simulink model "DA40_Flight_Model"  (R2023a)
settings: Solver=FixedStepAuto  StartTime=Start_Time  StopTime=End_Time  FixedStep=Time_Step  RelTol=1e-3
undefined symbols (not defined in the file or in its folder): BSFC_LUT, dayofyear, Earth, Initial_X, lookaheadDist, PowerFactor_LUT, STGeometry, Vehicle, waypoints, WGS84
libraries: slpidlib x8, simulink_extras x3, aerolibatmos2 x2, mspsensorlib x2, aerolibtransform2 x2, simulink x1, aerolibwind2 x1, uavalgslib x1
(part 1 of 3)
settings Model: Creator=izc0018  LastModifiedBy=noahm
settings DebuggingCC: AlgebraicLoopMsg=none  UnconnectedInputMsg=warning  UnconnectedOutputMsg=warning  UnconnectedLineMsg=warning
settings HardwareCC: ProdBitPerLong=64  ProdLargestAtomicFloat=None  ProdHWDeviceType=AMD->Athlon 64
settings ModelReferenceCC: EnableRefExpFcnMdlSchedulingChecks=on  ModelReferenceMinAlgLoopOccurrences=on
settings RTWCC: DLArmComputeVersion=19.05

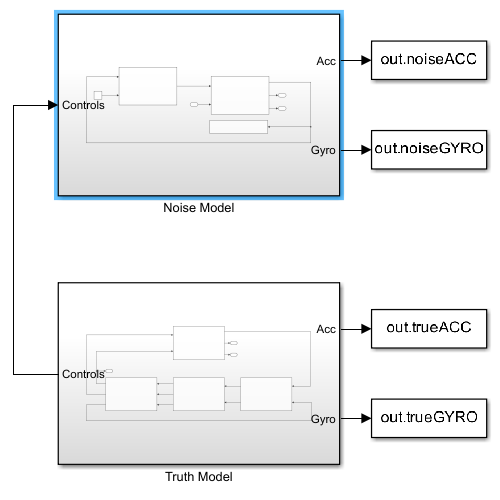
[thumbnail: Simulink's stored preview of the top-level diagram]
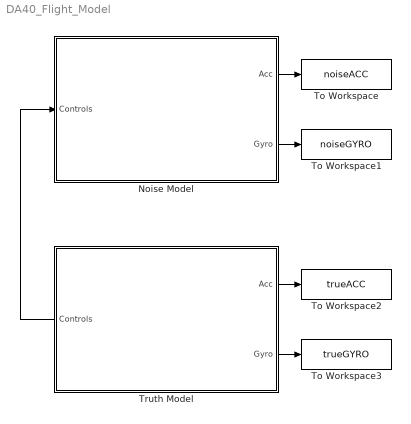
== system DA40_Flight_Model ==
  Noise Model : Subsystem
  To Workspace : ToWorkspace  VariableName=noiseACC  SaveFormat=Timeseries  SampleTime=-1
  To Workspace1 : ToWorkspace  VariableName=noiseGYRO  SaveFormat=Timeseries  SampleTime=-1
  To Workspace2 : ToWorkspace  VariableName=trueACC  SaveFormat=Timeseries  SampleTime=-1
  To Workspace3 : ToWorkspace  VariableName=trueGYRO  SaveFormat=Timeseries  SampleTime=-1
  Truth Model : Subsystem
      settings: PortSchema="{\"entries\":[{\"content\":{\"sides\":[{\"content\":{\"connectorIds\":[\"Out3\"]},\"type\":\"ConnectorPlacement.EquallySpacedRectSide\",\"uuid\":\"8eb98788-9771-4626-a3f5-af2a13caf3fb\"},{\"content\":{\"connectorIds\":[\"Out1\",\"Out2\"],\"side\":\"RIGHT\"},\"type\":\"ConnectorPlacement.EquallySpacedRectSide\",\"uuid\":\"345bd972-994d-44f9-8c5e-03b63b24e0ec\"},{\"content\":{\"side\":\"TOP\"},\"type\":\"ConnectorPlacement.EquallySpacedRectSide\",\"uuid\":\"1da6d2e0-f9fd-4d97-b889-7f9e1c209230\"}]},\"type\":\"ConnectorPlacement.EquallySpacedConnector\",\"uuid\":\"7d2beb0e-411b-47ae-aba6-e2acf08d65c2\"}],\"packageUris\":[\"http://schema.mathworks.com/mf0/Connector/R2020b\"],\"version\":\"1.0\"}"
  wires:
  Truth Model/3(Controls) -> Noise Model/1(Controls)
  Noise Model/1(Acc) -> To Workspace/1
  Noise Model/2(Gyro) -> To Workspace1/1
  Truth Model/1(Acc) -> To Workspace2/1
  Truth Model/2(Gyro) -> To Workspace3/1

== system DA40_Flight_Model/Noise Model ==
  Controls : Inport
  Band-Limited White Noise3 : simulink/Sources/Band-Limited White Noise  Cov=500  Ts=30  seed=1
  Environment : Subsystem
  Navigation : Subsystem
  Send To Workspace : Subsystem
  Acc : Outport
  Gyro : Outport  Port=2
  wires:
  Environment/1(Atmos) -> Navigation/1(Atmosphere)
  Navigation/1(States) -> Environment/1(States), Send To Workspace/1(States)
  Band-Limited White Noise3/1 -> Environment/2(Wind Model)
  Controls/1 -> Navigation/2(Controls)
  Navigation/2(Acc) -> Acc/1
  Navigation/3(Gyro) -> Gyro/1

== system DA40_Flight_Model/Truth Model ==
  Control : Subsystem
  Environment : Subsystem
  Guidance : Subsystem
  Navigation1 : Subsystem
  Acc : Outport
  Gyro : Outport  Port=2
  Controls : Outport  Port=3
  wires:
  Control/1(Controls) -> Navigation1/2(Controls), Controls/1
  Guidance/1(Commands) -> Control/1(Commands)
  Guidance/2(States Out) -> Control/2(States)
  Guidance/3(Atmos) -> Control/3(Atmos)
  Environment/1(States Out) -> Guidance/1(States)
  Environment/2(Atmos) -> Guidance/2(Atmosphere)
  Control/3(LLA) -> Environment/2(LLA)
  Control/2(Atmosphere) -> Navigation1/1(Atmosphere)
  Navigation1/1(States) -> Environment/1(States)
  Navigation1/2(Acc) -> Acc/1
  Navigation1/3(Gyro) -> Gyro/1

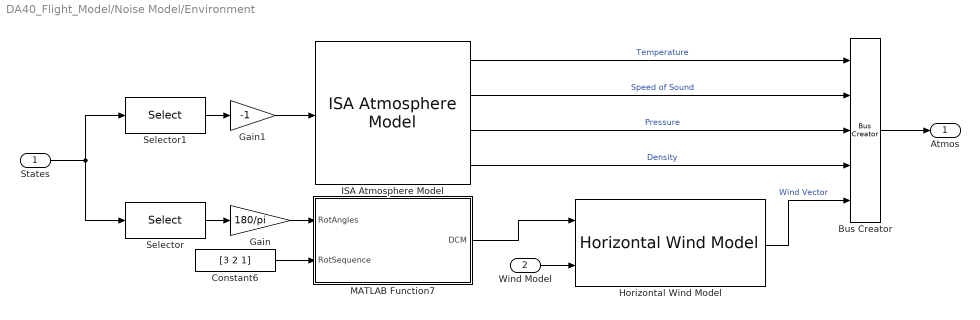
== system DA40_Flight_Model/Noise Model/Environment ==
  States : Inport
  Wind Model : Inport  Port=2
  Bus Creator : BusCreator  Inputs=5
  Constant6 : Constant  Value=[3 2 1]
  Gain : Gain  Gain=180/pi
  Gain1 : Gain  Gain=-1
  Horizontal Wind Model : aerolibwind2/Horizontal Wind Model  units=Metric (MKS)  Vw_source=External  Vwind=0  W_source=Internal  Wdeg=0
  ISA Atmosphere Model : aerolibatmos2/ISA Atmosphere Model  custom=off  g=9.80665  gamma=1.4  R=287.0531  L=0.0065  h_trop=11000  h_strat=20000  rho0=1.225  P0=101325  T0=288.15  h0=0
  MATLAB Function7 : MATLAB Function  TreatAsAtomicUnit=on
  Selector : Selector  InputPortWidth=12  IndexOptions=Index vector (dialog)  Indices=[10 11 12]  OutputSizes=1
  Selector1 : Selector  InputPortWidth=12  IndexOptions=Index vector (dialog)  Indices=[9]  OutputSizes=1
  Atmos : Outport
  wires:
  MATLAB Function7/1(DCM) -> Horizontal Wind Model/1
  States/1 -> Selector/1, Selector1/1
  Selector1/1 -> Gain1/1
  ISA Atmosphere Model/2 -> Bus Creator/2  "Speed of Sound"
  ISA Atmosphere Model/3 -> Bus Creator/3  "Pressure"
  Bus Creator/1 -> Atmos/1
  Selector/1 -> Gain/1
  ISA Atmosphere Model/1 -> Bus Creator/1  "Temperature"
  Gain/1 -> MATLAB Function7/1(RotAngles)
  ISA Atmosphere Model/4 -> Bus Creator/4  "Density"
  Constant6/1 -> MATLAB Function7/2(RotSequence)
  Horizontal Wind Model/1 -> Bus Creator/5  "Wind Vector"
  Gain1/1 -> ISA Atmosphere Model/1
  Wind Model/1 -> Horizontal Wind Model/2

== system DA40_Flight_Model/Noise Model/Navigation ==
  Atmosphere : Inport
  Controls : Inport  Port=2
  Constant1 : Constant  Value=Vehicle.MassProp.Mass
  DA-40 Equations of Motion : Subsystem
  Flight Mechanics and Systems Models : Subsystem
  States : Outport
  Acc : Outport  Port=2
  Gyro : Outport  Port=3
  wires:
  Flight Mechanics and Systems Models/1(Fb) -> DA-40 Equations of Motion/1(Fb [lb])
  Flight Mechanics and Systems Models/2(Mb) -> DA-40 Equations of Motion/2(Mb [lb-ft])
  Controls/1 -> Flight Mechanics and Systems Models/2(Control Commands)
  Atmosphere/1 -> Flight Mechanics and Systems Models/1(Atmosphere)
  Constant1/1 -> DA-40 Equations of Motion/3(Mass Properties)
  DA-40 Equations of Motion/3(States) -> States/1, Flight Mechanics and Systems Models/3(States)
  DA-40 Equations of Motion/1(Acc) -> Acc/1
  DA-40 Equations of Motion/2(Gyro) -> Gyro/1

== system DA40_Flight_Model/Noise Model/Send To Workspace ==
  States : Inport
  Constant : Constant  Value=0
  Demux : Demux  Outputs=2
  Flat Earth to LLA : aerolibtransform2/Flat Earth to LLA  units=Metric (MKS)  ptype=Earth (WGS84)  F=1/298.257223563  R=6378137  refPosPort=off  LL0=refLLA  psi=0
  Selector1 : Selector  InputPortWidth=12  IndexOptions=Index vector (dialog)  Indices=[7:9]  OutputSizes=1
  To Workspace1 : ToWorkspace  VariableName=noiseLONG  SampleTime=-1
  To Workspace2 : ToWorkspace  VariableName=noiseALT  SampleTime=-1
  To Workspace6 : ToWorkspace  VariableName=noiseLAT  SampleTime=-1
  wires:
  States/1 -> Selector1/1
  Selector1/1 -> Flat Earth to LLA/1
  Constant/1 -> Flat Earth to LLA/2
  Flat Earth to LLA/2 -> To Workspace2/1
  Flat Earth to LLA/1 -> Demux/1
  Demux/1 -> To Workspace6/1
  Demux/2 -> To Workspace1/1

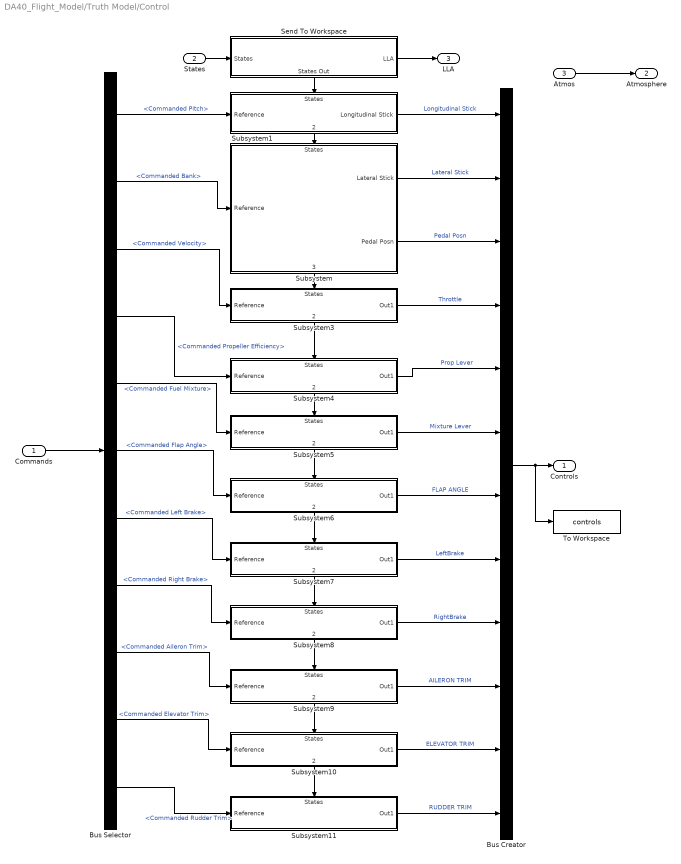
== system DA40_Flight_Model/Truth Model/Control ==
  Commands : Inport
  States : Inport  Port=2
  Atmos : Inport  Port=3
  Bus Creator : BusCreator  Inputs=12
  Bus Selector : BusSelector  OutputSignals=Commanded Pitch,Commanded Bank,Commanded Velocity,Commanded Propeller Efficiency,Commanded Fuel Mixture,Commanded Flap Angle,Commanded Left Brake,Commanded Right Brake,Commanded Aileron Trim,Commanded Elevator Trim,Commanded Rudder Trim
  Send To Workspace : Subsystem
      settings: PortSchema="{\"entries\":[{\"content\":{\"sides\":[{\"content\":{\"connectorIds\":[\"In1\"]},\"type\":\"ConnectorPlacement.EquallySpacedRectSide\",\"uuid\":\"f8d70518-feba-4467-9144-e72499141e10\"},{\"content\":{\"connectorIds\":[\"Out1\"],\"side\":\"RIGHT\"},\"type\":\"ConnectorPlacement.EquallySpacedRectSide\",\"uuid\":\"0d837ca8-6650-40ee-933a-3521e14176de\"},{\"content\":{\"side\":\"TOP\"},\"type\":\"ConnectorPlacement.EquallySpacedRectSide\",\"uuid\":\"54f7b60b-7724-46f0-8f38-219401d515c7\"},{\"content\":{\"connectorIds\":[\"Out2\"],\"side\":\"BOTTOM\"},\"type\":\"ConnectorPlacement.EquallySpacedRectSide\",\"uuid\":\"f1e71b5c-4796-4085-9245-75f71ccb39d6\"}]},\"type\":\"ConnectorPlacement.EquallySpacedConnector\",\"uuid\":\"946e06f8-2adb-45c5-9153-0b4b2f8d0bb6\"}],\"packageUris\":[\"http://schema.mathworks.com/mf0/Connector/R2020b\"],\"version\":\"1.0\"}"
  Subsystem : Subsystem
      settings: PortSchema="{\"entries\":[{\"content\":{\"sides\":[{\"content\":{\"connectorIds\":[\"In1\"]},\"type\":\"ConnectorPlacement.EquallySpacedRectSide\",\"uuid\":\"5ea7349d-baf6-49c5-809d-4b912ce56d76\"},{\"content\":{\"connectorIds\":[\"Out1\",\"Out2\"],\"side\":\"RIGHT\"},\"type\":\"ConnectorPlacement.EquallySpacedRectSide\",\"uuid\":\"ab3ceec7-e245-42b0-9eb8-e3a68951e219\"},{\"content\":{\"connectorIds\":[\"In2\"],\"side\":\"TOP\"},\"type\":\"ConnectorPlacement.EquallySpacedRectSide\",\"uuid\":\"18178c43-0035-4aec-a3ba-011af3830f5c\"},{\"content\":{\"connectorIds\":[\"Out3\"],\"side\":\"BOTTOM\"},\"type\":\"ConnectorPlacement.EquallySpacedRectSide\",\"uuid\":\"88476787-2df8-4308-98f2-16231590cef9\"}]},\"type\":\"ConnectorPlacement.EquallySpacedConnector\",\"uuid\":\"0f7476f8-a4e6-4d2f-9698-249fd1b1cc90\"}],\"packageUris\":[\"http://schema.mathworks.com/mf0/Connector/R2020b\"],\"version\":\"1.0\"}"
  Subsystem1 : Subsystem
      settings: PortSchema="{\"entries\":[{\"content\":{\"sides\":[{\"content\":{\"connectorIds\":[\"In1\"]},\"type\":\"ConnectorPlacement.EquallySpacedRectSide\",\"uuid\":\"df1e81ab-d97f-43f0-8cd1-ba06c25288e8\"},{\"content\":{\"connectorIds\":[\"Out1\"],\"side\":\"RIGHT\"},\"type\":\"ConnectorPlacement.EquallySpacedRectSide\",\"uuid\":\"fe7f65be-8a13-42ab-8ffa-afe418a633fa\"},{\"content\":{\"connectorIds\":[\"In2\"],\"side\":\"TOP\"},\"type\":\"ConnectorPlacement.EquallySpacedRectSide\",\"uuid\":\"4762097a-1dfd-4646-aeb3-678774417eb9\"},{\"content\":{\"connectorIds\":[\"Out2\"],\"side\":\"BOTTOM\"},\"type\":\"ConnectorPlacement.EquallySpacedRectSide\",\"uuid\":\"338e28fc-4594-4f48-8379-f1c16de78061\"}]},\"type\":\"ConnectorPlacement.EquallySpacedConnector\",\"uuid\":\"e1e6a329-5243-44ef-b6a4-a2802fff17f2\"}],\"packageUris\":[\"http://schema.mathworks.com/mf0/Connector/R2020b\"],\"version\":\"1.0\"}"
  Subsystem10 : Subsystem
      settings: PortSchema="{\"entries\":[{\"content\":{\"sides\":[{\"content\":{\"connectorIds\":[\"In1\"]},\"type\":\"ConnectorPlacement.EquallySpacedRectSide\",\"uuid\":\"df1e81ab-d97f-43f0-8cd1-ba06c25288e8\"},{\"content\":{\"connectorIds\":[\"Out1\"],\"side\":\"RIGHT\"},\"type\":\"ConnectorPlacement.EquallySpacedRectSide\",\"uuid\":\"fe7f65be-8a13-42ab-8ffa-afe418a633fa\"},{\"content\":{\"connectorIds\":[\"In2\"],\"side\":\"TOP\"},\"type\":\"ConnectorPlacement.EquallySpacedRectSide\",\"uuid\":\"4762097a-1dfd-4646-aeb3-678774417eb9\"},{\"content\":{\"connectorIds\":[\"Out2\"],\"side\":\"BOTTOM\"},\"type\":\"ConnectorPlacement.EquallySpacedRectSide\",\"uuid\":\"ca232b1a-28ac-4e7a-b8a6-76103b2c6113\"}]},\"type\":\"ConnectorPlacement.EquallySpacedConnector\",\"uuid\":\"e1e6a329-5243-44ef-b6a4-a2802fff17f2\"}],\"packageUris\":[\"http://schema.mathworks.com/mf0/Connector/R2020b\"],\"version\":\"1.0\"}"
  Subsystem11 : Subsystem
      settings: PortSchema="{\"entries\":[{\"content\":{\"sides\":[{\"content\":{\"connectorIds\":[\"In1\"]},\"type\":\"ConnectorPlacement.EquallySpacedRectSide\",\"uuid\":\"df1e81ab-d97f-43f0-8cd1-ba06c25288e8\"},{\"content\":{\"connectorIds\":[\"Out1\"],\"side\":\"RIGHT\"},\"type\":\"ConnectorPlacement.EquallySpacedRectSide\",\"uuid\":\"fe7f65be-8a13-42ab-8ffa-afe418a633fa\"},{\"content\":{\"connectorIds\":[\"In2\"],\"side\":\"TOP\"},\"type\":\"ConnectorPlacement.EquallySpacedRectSide\",\"uuid\":\"4762097a-1dfd-4646-aeb3-678774417eb9\"}]},\"type\":\"ConnectorPlacement.EquallySpacedConnector\",\"uuid\":\"e1e6a329-5243-44ef-b6a4-a2802fff17f2\"}],\"packageUris\":[\"http://schema.mathworks.com/mf0/Connector/R2020b\"],\"version\":\"1.0\"}"
  Subsystem3 : Subsystem
      settings: PortSchema="{\"entries\":[{\"content\":{\"sides\":[{\"content\":{\"connectorIds\":[\"In1\"]},\"type\":\"ConnectorPlacement.EquallySpacedRectSide\",\"uuid\":\"df1e81ab-d97f-43f0-8cd1-ba06c25288e8\"},{\"content\":{\"connectorIds\":[\"Out1\"],\"side\":\"RIGHT\"},\"type\":\"ConnectorPlacement.EquallySpacedRectSide\",\"uuid\":\"fe7f65be-8a13-42ab-8ffa-afe418a633fa\"},{\"content\":{\"connectorIds\":[\"In2\"],\"side\":\"TOP\"},\"type\":\"ConnectorPlacement.EquallySpacedRectSide\",\"uuid\":\"4762097a-1dfd-4646-aeb3-678774417eb9\"},{\"content\":{\"connectorIds\":[\"Out2\"],\"side\":\"BOTTOM\"},\"type\":\"ConnectorPlacement.EquallySpacedRectSide\",\"uuid\":\"eb7acd08-7b98-4b28-a61a-3ca4385205ec\"}]},\"type\":\"ConnectorPlacement.EquallySpacedConnector\",\"uuid\":\"e1e6a329-5243-44ef-b6a4-a2802fff17f2\"}],\"packageUris\":[\"http://schema.mathworks.com/mf0/Connector/R2020b\"],\"version\":\"1.0\"}"
  Subsystem4 : Subsystem
      settings: PortSchema="{\"entries\":[{\"content\":{\"sides\":[{\"content\":{\"connectorIds\":[\"In1\"]},\"type\":\"ConnectorPlacement.EquallySpacedRectSide\",\"uuid\":\"df1e81ab-d97f-43f0-8cd1-ba06c25288e8\"},{\"content\":{\"connectorIds\":[\"Out1\"],\"side\":\"RIGHT\"},\"type\":\"ConnectorPlacement.EquallySpacedRectSide\",\"uuid\":\"fe7f65be-8a13-42ab-8ffa-afe418a633fa\"},{\"content\":{\"connectorIds\":[\"In2\"],\"side\":\"TOP\"},\"type\":\"ConnectorPlacement.EquallySpacedRectSide\",\"uuid\":\"4762097a-1dfd-4646-aeb3-678774417eb9\"},{\"content\":{\"connectorIds\":[\"Out2\"],\"side\":\"BOTTOM\"},\"type\":\"ConnectorPlacement.EquallySpacedRectSide\",\"uuid\":\"aca1bd27-9370-4c71-9435-0c269f9a438b\"}]},\"type\":\"ConnectorPlacement.EquallySpacedConnector\",\"uuid\":\"e1e6a329-5243-44ef-b6a4-a2802fff17f2\"}],\"packageUris\":[\"http://schema.mathworks.com/mf0/Connector/R2020b\"],\"version\":\"1.0\"}"
  Subsystem5 : Subsystem
      settings: PortSchema="{\"entries\":[{\"content\":{\"sides\":[{\"content\":{\"connectorIds\":[\"In1\"]},\"type\":\"ConnectorPlacement.EquallySpacedRectSide\",\"uuid\":\"df1e81ab-d97f-43f0-8cd1-ba06c25288e8\"},{\"content\":{\"connectorIds\":[\"Out1\"],\"side\":\"RIGHT\"},\"type\":\"ConnectorPlacement.EquallySpacedRectSide\",\"uuid\":\"fe7f65be-8a13-42ab-8ffa-afe418a633fa\"},{\"content\":{\"connectorIds\":[\"In2\"],\"side\":\"TOP\"},\"type\":\"ConnectorPlacement.EquallySpacedRectSide\",\"uuid\":\"4762097a-1dfd-4646-aeb3-678774417eb9\"},{\"content\":{\"connectorIds\":[\"Out2\"],\"side\":\"BOTTOM\"},\"type\":\"ConnectorPlacement.EquallySpacedRectSide\",\"uuid\":\"e3132084-5e8e-4693-9249-2c258902bcf1\"}]},\"type\":\"ConnectorPlacement.EquallySpacedConnector\",\"uuid\":\"e1e6a329-5243-44ef-b6a4-a2802fff17f2\"}],\"packageUris\":[\"http://schema.mathworks.com/mf0/Connector/R2020b\"],\"version\":\"1.0\"}"
  Subsystem6 : Subsystem
      settings: PortSchema="{\"entries\":[{\"content\":{\"sides\":[{\"content\":{\"connectorIds\":[\"In1\"]},\"type\":\"ConnectorPlacement.EquallySpacedRectSide\",\"uuid\":\"df1e81ab-d97f-43f0-8cd1-ba06c25288e8\"},{\"content\":{\"connectorIds\":[\"Out1\"],\"side\":\"RIGHT\"},\"type\":\"ConnectorPlacement.EquallySpacedRectSide\",\"uuid\":\"fe7f65be-8a13-42ab-8ffa-afe418a633fa\"},{\"content\":{\"connectorIds\":[\"In2\"],\"side\":\"TOP\"},\"type\":\"ConnectorPlacement.EquallySpacedRectSide\",\"uuid\":\"4762097a-1dfd-4646-aeb3-678774417eb9\"},{\"content\":{\"connectorIds\":[\"Out2\"],\"side\":\"BOTTOM\"},\"type\":\"ConnectorPlacement.EquallySpacedRectSide\",\"uuid\":\"44b8b4cf-3de4-40e9-9bc3-b7b2ed15b9c4\"}]},\"type\":\"ConnectorPlacement.EquallySpacedConnector\",\"uuid\":\"e1e6a329-5243-44ef-b6a4-a2802fff17f2\"}],\"packageUris\":[\"http://schema.mathworks.com/mf0/Connector/R2020b\"],\"version\":\"1.0\"}"
  Subsystem7 : Subsystem
      settings: PortSchema="{\"entries\":[{\"content\":{\"sides\":[{\"content\":{\"connectorIds\":[\"In1\"]},\"type\":\"ConnectorPlacement.EquallySpacedRectSide\",\"uuid\":\"df1e81ab-d97f-43f0-8cd1-ba06c25288e8\"},{\"content\":{\"connectorIds\":[\"Out1\"],\"side\":\"RIGHT\"},\"type\":\"ConnectorPlacement.EquallySpacedRectSide\",\"uuid\":\"fe7f65be-8a13-42ab-8ffa-afe418a633fa\"},{\"content\":{\"connectorIds\":[\"In2\"],\"side\":\"TOP\"},\"type\":\"ConnectorPlacement.EquallySpacedRectSide\",\"uuid\":\"4762097a-1dfd-4646-aeb3-678774417eb9\"},{\"content\":{\"connectorIds\":[\"Out2\"],\"side\":\"BOTTOM\"},\"type\":\"ConnectorPlacement.EquallySpacedRectSide\",\"uuid\":\"4aea28e3-05ae-492c-9523-17787d8052fd\"}]},\"type\":\"ConnectorPlacement.EquallySpacedConnector\",\"uuid\":\"e1e6a329-5243-44ef-b6a4-a2802fff17f2\"}],\"packageUris\":[\"http://schema.mathworks.com/mf0/Connector/R2020b\"],\"version\":\"1.0\"}"
  Subsystem8 : Subsystem
      settings: PortSchema="{\"entries\":[{\"content\":{\"sides\":[{\"content\":{\"connectorIds\":[\"In1\"]},\"type\":\"ConnectorPlacement.EquallySpacedRectSide\",\"uuid\":\"df1e81ab-d97f-43f0-8cd1-ba06c25288e8\"},{\"content\":{\"connectorIds\":[\"Out1\"],\"side\":\"RIGHT\"},\"type\":\"ConnectorPlacement.EquallySpacedRectSide\",\"uuid\":\"fe7f65be-8a13-42ab-8ffa-afe418a633fa\"},{\"content\":{\"connectorIds\":[\"In2\"],\"side\":\"TOP\"},\"type\":\"ConnectorPlacement.EquallySpacedRectSide\",\"uuid\":\"4762097a-1dfd-4646-aeb3-678774417eb9\"},{\"content\":{\"connectorIds\":[\"Out2\"],\"side\":\"BOTTOM\"},\"type\":\"ConnectorPlacement.EquallySpacedRectSide\",\"uuid\":\"60b425fe-182c-41c2-bc4c-aa97cb3d7ccf\"}]},\"type\":\"ConnectorPlacement.EquallySpacedConnector\",\"uuid\":\"e1e6a329-5243-44ef-b6a4-a2802fff17f2\"}],\"packageUris\":[\"http://schema.mathworks.com/mf0/Connector/R2020b\"],\"version\":\"1.0\"}"
  Subsystem9 : Subsystem
      settings: PortSchema="{\"entries\":[{\"content\":{\"sides\":[{\"content\":{\"connectorIds\":[\"In1\"]},\"type\":\"ConnectorPlacement.EquallySpacedRectSide\",\"uuid\":\"df1e81ab-d97f-43f0-8cd1-ba06c25288e8\"},{\"content\":{\"connectorIds\":[\"Out1\"],\"side\":\"RIGHT\"},\"type\":\"ConnectorPlacement.EquallySpacedRectSide\",\"uuid\":\"fe7f65be-8a13-42ab-8ffa-afe418a633fa\"},{\"content\":{\"connectorIds\":[\"In2\"],\"side\":\"TOP\"},\"type\":\"ConnectorPlacement.EquallySpacedRectSide\",\"uuid\":\"4762097a-1dfd-4646-aeb3-678774417eb9\"},{\"content\":{\"connectorIds\":[\"Out2\"],\"side\":\"BOTTOM\"},\"type\":\"ConnectorPlacement.EquallySpacedRectSide\",\"uuid\":\"88e2b07d-9cf7-412b-8368-04827ebf702b\"}]},\"type\":\"ConnectorPlacement.EquallySpacedConnector\",\"uuid\":\"e1e6a329-5243-44ef-b6a4-a2802fff17f2\"}],\"packageUris\":[\"http://schema.mathworks.com/mf0/Connector/R2020b\"],\"version\":\"1.0\"}"
  To Workspace : ToWorkspace  VariableName=controls  SampleTime=-1
      settings: Save2DSignal=2-D array (concatenate along first dimension)
  Controls : Outport
  Atmosphere : Outport  Port=2
  LLA : Outport  Port=3
  wires:
  Subsystem11/1(Out1) -> Bus Creator/12  "RUDDER TRIM"
  Subsystem9/1(Out1) -> Bus Creator/10  "AILERON TRIM"
  Subsystem1/1(Longitudinal Stick) -> Bus Creator/1  "Longitudinal Stick"
  Subsystem/1(Lateral Stick) -> Bus Creator/2  "Lateral Stick"
  Subsystem6/1(Out1) -> Bus Creator/7  "FLAP ANGLE"
  Subsystem5/1(Out1) -> Bus Creator/6  "Mixture Lever"
  Subsystem3/1(Out1) -> Bus Creator/4  "Throttle"
  Subsystem8/1(Out1) -> Bus Creator/9  "RightBrake"
  Subsystem/2(Pedal Posn) -> Bus Creator/3  "Pedal Posn"
  Subsystem4/1(Out1) -> Bus Creator/5  "Prop Lever"
  Subsystem7/1(Out1) -> Bus Creator/8  "LeftBrake"
  Subsystem10/1(Out1) -> Bus Creator/11  "ELEVATOR TRIM"
  Bus Creator/1 -> To Workspace/1, Controls/1
  Commands/1 -> Bus Selector/1
  Bus Selector/11 -> Subsystem11/1(Reference)  "<Commanded Rudder Trim>"
  Bus Selector/10 -> Subsystem10/1(Reference)  "<Commanded Elevator Trim>"
  Bus Selector/9 -> Subsystem9/1(Reference)  "<Commanded Aileron Trim>"
  Bus Selector/8 -> Subsystem8/1(Reference)  "<Commanded Right Brake>"
  Bus Selector/7 -> Subsystem7/1(Reference)  "<Commanded Left Brake>"
  Bus Selector/6 -> Subsystem6/1(Reference)  "<Commanded Flap Angle>"
  Bus Selector/5 -> Subsystem5/1(Reference)  "<Commanded Fuel Mixture>"
  Bus Selector/4 -> Subsystem4/1(Reference)  "<Commanded Propeller Efficiency>"
  Bus Selector/3 -> Subsystem3/1(Reference)  "<Commanded Velocity>"
  Bus Selector/1 -> Subsystem1/1(Reference)  "<Commanded Pitch>"
  Bus Selector/2 -> Subsystem/1(Reference)  "<Commanded Bank>"
  States/1 -> Send To Workspace/1(States)
  Send To Workspace/2(States Out) -> Subsystem1/2(States)
  Subsystem6/2(" ") -> Subsystem7/2(States)
  Subsystem9/2(" ") -> Subsystem10/2(States)
  Subsystem3/2(" ") -> Subsystem4/2(States)
  Subsystem/3(" ") -> Subsystem3/2(States)
  Subsystem1/2(" ") -> Subsystem/2(States)
  Subsystem7/2(" ") -> Subsystem8/2(States)
  Subsystem8/2(" ") -> Subsystem9/2(States)
  Subsystem5/2(" ") -> Subsystem6/2(States)
  Subsystem4/2(" ") -> Subsystem5/2(States)
  Subsystem10/2(" ") -> Subsystem11/2(States)
  Atmos/1 -> Atmosphere/1
  Send To Workspace/1(LLA) -> LLA/1

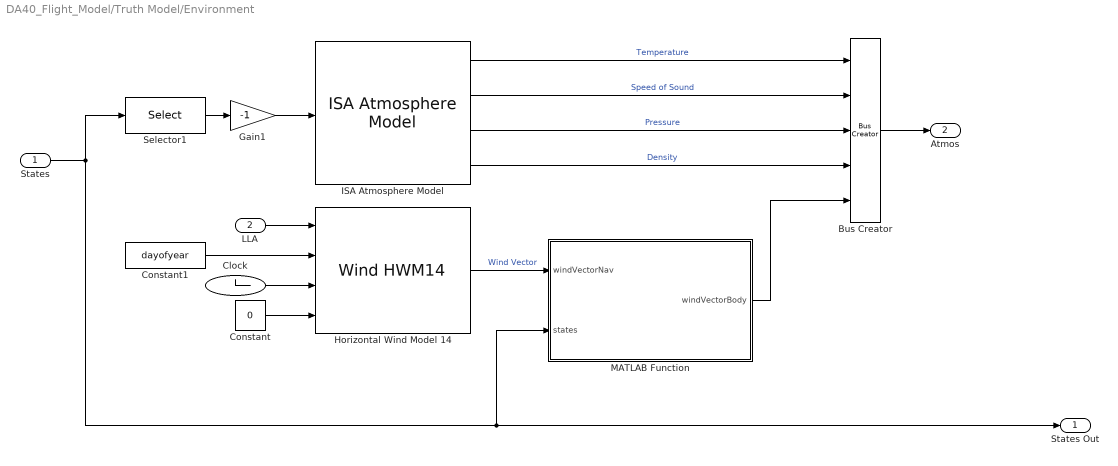
== system DA40_Flight_Model/Truth Model/Environment ==
  States : Inport
  LLA : Inport  Port=2
  Bus Creator : BusCreator  Inputs=5
  Clock : Clock
  Constant : Constant  Value=0
  Constant1 : Constant  Value=dayofyear
  Gain1 : Gain  Gain=-1
  Horizontal Wind Model 14 : WindHWM14  model=Total
  ISA Atmosphere Model : aerolibatmos2/ISA Atmosphere Model  custom=off  g=9.80665  gamma=1.4  R=287.0531  L=0.0065  h_trop=11000  h_strat=20000  rho0=1.225  P0=101325  T0=288.15  h0=0
  MATLAB Function : MATLAB Function  TreatAsAtomicUnit=on
  Selector1 : Selector  InputPortWidth=12  IndexOptions=Index vector (dialog)  Indices=[9]  OutputSizes=1
  States Out : Outport
  Atmos : Outport  Port=2
  wires:
  States/1 -> MATLAB Function/2(states), States Out/1, Selector1/1
  Selector1/1 -> Gain1/1
  ISA Atmosphere Model/2 -> Bus Creator/2  "Speed of Sound"
  ISA Atmosphere Model/3 -> Bus Creator/3  "Pressure"
  Bus Creator/1 -> Atmos/1
  ISA Atmosphere Model/1 -> Bus Creator/1  "Temperature"
  Gain1/1 -> ISA Atmosphere Model/1
  ISA Atmosphere Model/4 -> Bus Creator/4  "Density"
  LLA/1 -> Horizontal Wind Model 14/1
  Clock/1 -> Horizontal Wind Model 14/3
  Constant/1 -> Horizontal Wind Model 14/4
  Constant1/1 -> Horizontal Wind Model 14/2
  Horizontal Wind Model 14/1 -> MATLAB Function/1(windVectorNav)  "Wind Vector"
  MATLAB Function/1(windVectorBody) -> Bus Creator/5

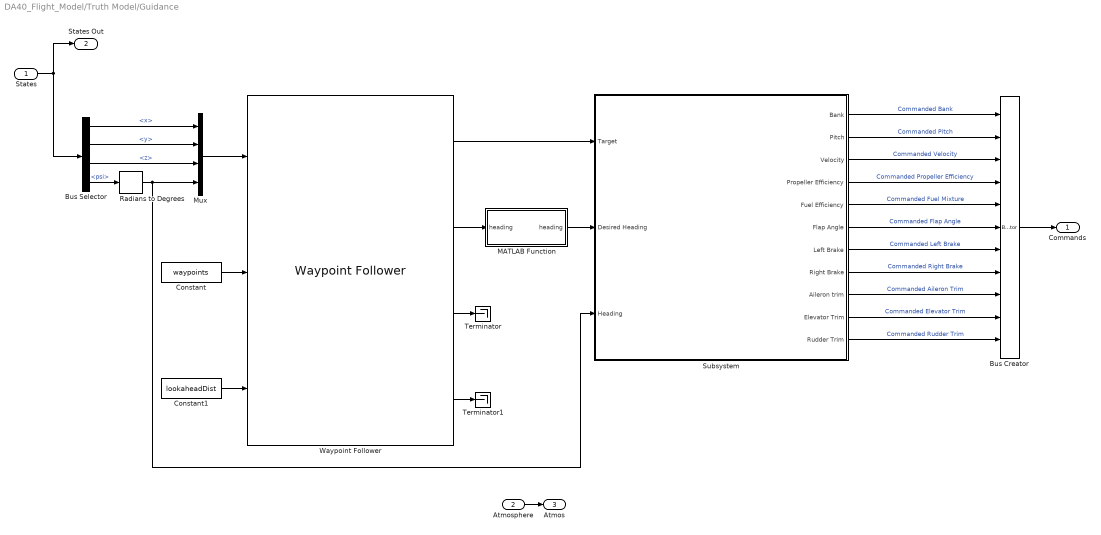
== system DA40_Flight_Model/Truth Model/Guidance ==
  States : Inport
  Atmosphere : Inport  Port=2
  Bus Creator : BusCreator  Inputs=11
  Bus Selector : BusSelector  OutputSignals=x,y,z,psi
  Constant : Constant  Value=waypoints
  Constant1 : Constant  Value=lookaheadDist
  MATLAB Function : MATLAB Function  TreatAsAtomicUnit=on
  Mux : Mux
  Radians to Degrees : simulink_extras/Transformations/Radians to Degrees
  Subsystem : Subsystem
  Terminator : Terminator
  Terminator1 : Terminator
  Waypoint Follower : uavalgslib/Waypoint Follower  UAVType=fixed-wing  StartFrom=first  TransitionRadiusSource=internal  TransitionRadius=10  MinLookaheadDistance=0.1  YawInput=off  ShowCrossTrackErrorOutput=off  ShowStatusOutput=off  SimulateUsing=Code generation
  Commands : Outport
  States Out : Outport  Port=2
  Atmos : Outport  Port=3
  wires:
  Bus Creator/1 -> Commands/1
  Subsystem/1(Bank) -> Bus Creator/1  "Commanded Bank"
  Subsystem/2(Pitch) -> Bus Creator/2  "Commanded Pitch"
  Subsystem/3(Velocity) -> Bus Creator/3  "Commanded Velocity"
  Subsystem/4(Propeller Efficiency) -> Bus Creator/4  "Commanded Propeller Efficiency"
  Subsystem/5(Fuel Efficiency) -> Bus Creator/5  "Commanded Fuel Mixture"
  Subsystem/6(Flap Angle) -> Bus Creator/6  "Commanded Flap Angle"
  Subsystem/7(Left Brake) -> Bus Creator/7  "Commanded Left Brake"
  Subsystem/8(Right Brake) -> Bus Creator/8  "Commanded Right Brake"
  Subsystem/9(Aileron trim) -> Bus Creator/9  "Commanded Aileron Trim"
  Subsystem/10(Elevator Trim) -> Bus Creator/10  "Commanded Elevator Trim"
  Subsystem/11(Rudder Trim) -> Bus Creator/11  "Commanded Rudder Trim"
  States/1 -> Bus Selector/1, States Out/1
  Waypoint Follower/3 -> Terminator/1
  Waypoint Follower/4 -> Terminator1/1
  Constant/1 -> Waypoint Follower/2
  Constant1/1 -> Waypoint Follower/3
  Mux/1 -> Waypoint Follower/1
  Bus Selector/1 -> Mux/1  "<x>"
  Bus Selector/2 -> Mux/2  "<y>"
  Bus Selector/3 -> Mux/3  "<z>"
  Waypoint Follower/2 -> MATLAB Function/1("heading ")
  Atmosphere/1 -> Atmos/1
  Waypoint Follower/1 -> Subsystem/1(Target)
  MATLAB Function/1(heading) -> Subsystem/2(Desired Heading)
  Radians to Degrees/1 -> Mux/4, Subsystem/3(Heading)
  Bus Selector/4 -> Radians to Degrees/1  "<psi>"

== system DA40_Flight_Model/Truth Model/Navigation1 ==
  Atmosphere : Inport
  Controls : Inport  Port=2
  Constant1 : Constant  Value=Vehicle.MassProp.Mass
  DA-40 Equations of Motion : Subsystem
  Flight Mechanics and Systems Models : Subsystem
  States : Outport
  Acc : Outport  Port=2
  Gyro : Outport  Port=3
  wires:
  Flight Mechanics and Systems Models/1(Fb) -> DA-40 Equations of Motion/1(Fb [lb])
  Flight Mechanics and Systems Models/2(Mb) -> DA-40 Equations of Motion/2(Mb [lb-ft])
  Controls/1 -> Flight Mechanics and Systems Models/2(Control Commands)
  Atmosphere/1 -> Flight Mechanics and Systems Models/1(Atmosphere)
  Constant1/1 -> DA-40 Equations of Motion/3(Mass Properties)
  DA-40 Equations of Motion/3(States) -> States/1, Flight Mechanics and Systems Models/3(States)
  DA-40 Equations of Motion/1(Acc) -> Acc/1
  DA-40 Equations of Motion/2(Gyro) -> Gyro/1

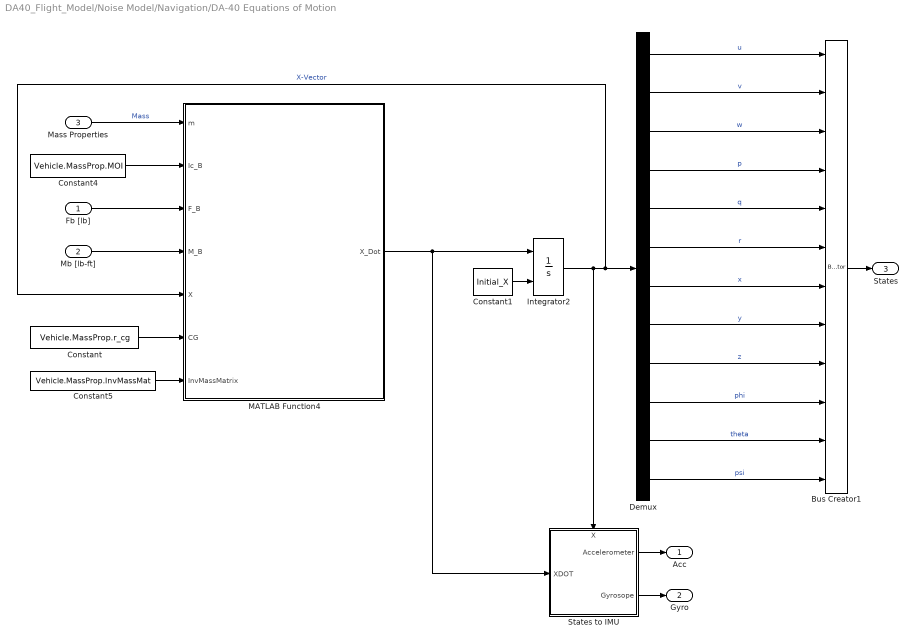
== system DA40_Flight_Model/Noise Model/Navigation/DA-40 Equations of Motion ==
  Fb [lb] : Inport
  Mb [lb-ft] : Inport  Port=2
  Mass Properties : Inport  Port=3
  Bus Creator1 : BusCreator  Inputs=12
  Constant : Constant  Value=Vehicle.MassProp.r_cg
  Constant1 : Constant  Value=Initial_X
  Constant4 : Constant  Value=Vehicle.MassProp.MOI  VectorParams1D=off
  Constant5 : Constant  Value=Vehicle.MassProp.InvMassMat
  Demux : Demux  Outputs=12
  Integrator2 : Integrator  InitialConditionSource=external
  MATLAB Function4 : MATLAB Function  TreatAsAtomicUnit=on
  States to IMU : Subsystem
      settings: PortSchema="{\"entries\":[{\"content\":{\"sides\":[{\"content\":{\"connectorIds\":[\"In1\"]},\"type\":\"ConnectorPlacement.EquallySpacedRectSide\",\"uuid\":\"70ccec87-9e5d-4668-bab7-5e3830192650\"},{\"content\":{\"connectorIds\":[\"Out1\",\"Out2\"],\"side\":\"RIGHT\"},\"type\":\"ConnectorPlacement.EquallySpacedRectSide\",\"uuid\":\"cc9275bd-5621-4491-a3fb-001b77b42a94\"},{\"content\":{\"connectorIds\":[\"In2\"],\"side\":\"TOP\"},\"type\":\"ConnectorPlacement.EquallySpacedRectSide\",\"uuid\":\"9fc04c5e-8168-4117-852d-b94be052fe47\"}]},\"type\":\"ConnectorPlacement.EquallySpacedConnector\",\"uuid\":\"901299e0-db58-4c82-bff1-da00e9d52dc5\"}],\"packageUris\":[\"http://schema.mathworks.com/mf0/Connector/R2020b\"],\"version\":\"1.0\"}"
  Acc : Outport
  Gyro : Outport  Port=2
  States : Outport  Port=3
  wires:
  Mb [lb-ft]/1 -> MATLAB Function4/4(M_B)
  Fb [lb]/1 -> MATLAB Function4/3(F_B)
  Mass Properties/1 -> MATLAB Function4/1(m)  "Mass"
  Constant4/1 -> MATLAB Function4/2(Ic_B)
  Constant1/1 -> Integrator2/2
  Integrator2/1 -> States to IMU/2(X), MATLAB Function4/5(X), Demux/1  "X-Vector"
  Constant/1 -> MATLAB Function4/6(CG)
  Constant5/1 -> MATLAB Function4/7(InvMassMatrix)
  Demux/1 -> Bus Creator1/1  "u"
  Demux/2 -> Bus Creator1/2  "v"
  Demux/3 -> Bus Creator1/3  "w"
  Demux/4 -> Bus Creator1/4  "p"
  Demux/5 -> Bus Creator1/5  "q"
  Demux/6 -> Bus Creator1/6  "r"
  Demux/7 -> Bus Creator1/7  "x"
  Demux/8 -> Bus Creator1/8  "y"
  Demux/9 -> Bus Creator1/9  "z"
  Demux/10 -> Bus Creator1/10  "phi"
  Demux/11 -> Bus Creator1/11  "theta"
  Demux/12 -> Bus Creator1/12  "psi"
  MATLAB Function4/1(X_Dot) -> States to IMU/1(XDOT), Integrator2/1
  States to IMU/1(Accelerometer) -> Acc/1
  States to IMU/2(Gyrosope) -> Gyro/1
  Bus Creator1/1 -> States/1

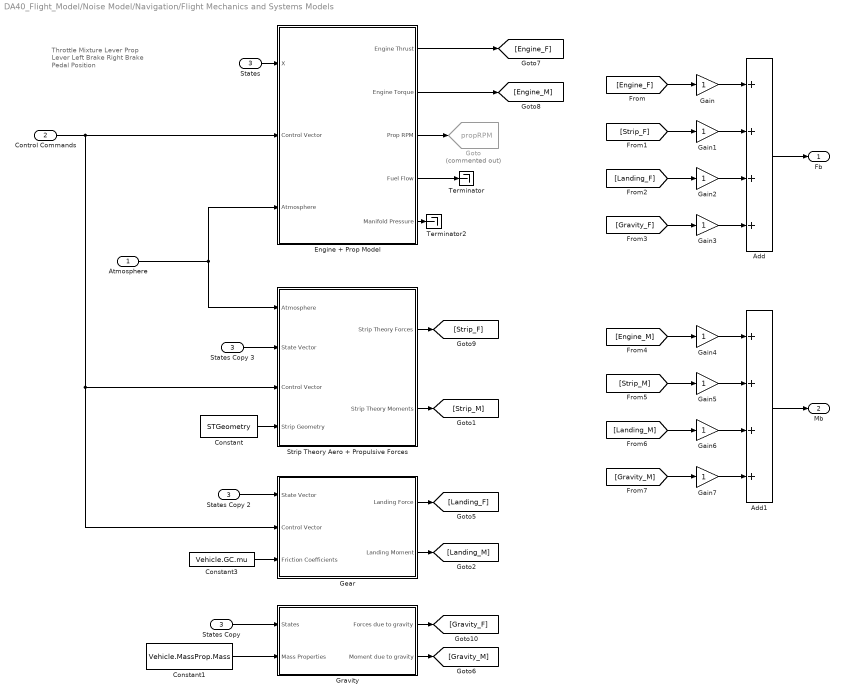
== system DA40_Flight_Model/Noise Model/Navigation/Flight Mechanics and Systems Models ==
  note: Throttle
      | Mixture Lever
      | Prop Lever
      | Left Brake
      | Right Brake
      | Pedal Position
  Atmosphere : Inport
  Control Commands : Inport  Port=2
  States : Inport  Port=3
  Add : Sum  Inputs=++++
  Add1 : Sum  Inputs=++++
  Constant : Constant  Value=STGeometry
  Constant1 : Constant  Value=Vehicle.MassProp.Mass
  Constant3 : Constant  Value=Vehicle.GC.mu
  Engine + Prop Model : Subsystem
  Gain{,1..7} (8 alike) : Gain
  Gear : Subsystem
  Goto : Goto  Commented=on  GotoTag=propRPM  TagVisibility=global
  Gravity : Subsystem
  States Copy : InportShadow  Port=3
  States Copy 2 : InportShadow  Port=3
  States Copy 3 : InportShadow  Port=3
  Strip Theory Aero + Propulsive Forces : Subsystem
  Terminator : Terminator
  Terminator2 : Terminator
  Fb : Outport
  Mb : Outport  Port=2
  wires:
  States/1 -> Engine + Prop Model/1(X)
  Constant1/1 -> Gravity/2(Mass Properties)
  Constant/1 -> Strip Theory Aero + Propulsive Forces/4(Strip Geometry)
  Engine + Prop Model/5(Manifold Pressure) -> Terminator2/1
  Engine + Prop Model/3(Prop RPM) -> Goto/1
  Constant3/1 -> Gear/3(Friction Coefficients)
  Add1/1 -> Mb/1
  States Copy/1 -> Gravity/1(States)
  States Copy 2/1 -> Gear/1(State Vector)
  States Copy 3/1 -> Strip Theory Aero + Propulsive Forces/2(State Vector)
  Control Commands/1 -> Strip Theory Aero + Propulsive Forces/3(Control Vector), Gear/2(Control Vector), Engine + Prop Model/2(Control Vector)
  Engine + Prop Model/2(Engine Torque) -> [Engine_M]
  Strip Theory Aero + Propulsive Forces/2(Strip Theory Moments) -> [Strip_M]
  Gear/2(Landing Moment) -> [Landing_M]
  Gravity/2(Moment due to gravity) -> [Gravity_M]
  Gravity/1(Forces due to gravity) -> [Gravity_F]
  Gear/1(Landing Force) -> [Landing_F]
  Strip Theory Aero + Propulsive Forces/1(Strip Theory Forces) -> [Strip_F]
  Engine + Prop Model/1(Engine Thrust) -> [Engine_F]
  Add/1 -> Fb/1
  [Engine_F] -> Gain/1
  [Strip_F] -> Gain1/1
  [Landing_F] -> Gain2/1
  [Gravity_F] -> Gain3/1
  [Engine_M] -> Gain4/1
  [Strip_M] -> Gain5/1
  [Landing_M] -> Gain6/1
  [Gravity_M] -> Gain7/1
  Gain/1 -> Add/1
  Gain1/1 -> Add/2
  Gain2/1 -> Add/3
  Gain3/1 -> Add/4
  Gain4/1 -> Add1/1
  Gain5/1 -> Add1/2
  Gain6/1 -> Add1/3
  Gain7/1 -> Add1/4
  Atmosphere/1 -> Strip Theory Aero + Propulsive Forces/1(Atmosphere), Engine + Prop Model/3(Atmosphere)
  Engine + Prop Model/4(Fuel Flow) -> Terminator/1

== system DA40_Flight_Model/Truth Model/Control/Send To Workspace ==
  States : Inport
  Constant : Constant  Value=0
  Demux : Demux  Outputs=2
  Flat Earth to LLA : aerolibtransform2/Flat Earth to LLA  units=Metric (MKS)  ptype=Earth (WGS84)  F=1/298.257223563  R=6378137  refPosPort=off  LL0=refLLA  psi=0
  Mux : Mux  Inputs=3
  Selector1 : Selector  InputPortWidth=12  IndexOptions=Index vector (dialog)  Indices=[7:9]  OutputSizes=1
  To Workspace1 : ToWorkspace  VariableName=trueLONG  SampleTime=-1
  To Workspace2 : ToWorkspace  VariableName=trueALT  SampleTime=-1
  To Workspace6 : ToWorkspace  VariableName=trueLAT  SampleTime=-1
  LLA : Outport
  States Out : Outport  Port=2
  wires:
  States/1 -> States Out/1, Selector1/1
  Selector1/1 -> Flat Earth to LLA/1
  Constant/1 -> Flat Earth to LLA/2
  Flat Earth to LLA/2 -> Mux/3, To Workspace2/1
  Flat Earth to LLA/1 -> Demux/1
  Demux/1 -> Mux/1, To Workspace6/1
  Demux/2 -> Mux/2, To Workspace1/1
  Mux/1 -> LLA/1

== system DA40_Flight_Model/Truth Model/Control/Subsystem ==
  Reference : Inport
  States : Inport  Port=2
  BANK HOLD PID : slpidlib/PID Controller (2DOF)  Controller=PID  Form=Parallel  TimeDomain=Continuous-time  UseExternalTs=off  SampleTime=-1  IntegratorMethod=Forward Euler  FilterMethod=Forward Euler  ControllerParametersSource=internal  P=0.107891692261891  I=0.133343747084316  UseKiTs=off  D=0.0171409705451499  N=25.8919437213056  UseFilter=on  b=0.548332573243903  c=0.00478750158934923  TunerSelectOption=Transfer Function Based (PID Tuner App)  InitialConditionSource=internal  InitialConditionForIntegrator=0  InitialConditionForFilter=0  DifferentiatorICPrevScaledInput=0  ExternalReset=none  TrackingMode=off  Kt=1  LimitOutput=on  SatLimitsSource=internal  UpperSaturationLimit=1  LowerSaturationLimit=-1  LinearizeAsGain=on  AntiWindupMode=clamping  Kb=1  LimitIntegrator=off  UpperIntegratorSaturationLimit=inf  LowerIntegratorSaturationLimit=-inf  POutMin=[]  POutMax=[]  IOutMin=[]  IOutMax=[]  DOutMin=[]  DOutMax=[]  NOutMin=[]  NOutMax=[]  bOutMin=[]  bOutMax=[]  cOutMin=[]  cOutMax=[]  SumOutMin=[]  SumOutMax=[]  SaturationOutMin=[]  SaturationOutMax=[]  PParamMin=[]  PParamMax=[]  IParamMin=[]  IParamMax=[]  DParamMin=[]  DParamMax=[]  NParamMin=[]  NParamMax=[]  bParamMin=[]  bParamMax=[]  cParamMin=[]  cParamMax=[]  KbParamMin=[]  KbParamMax=[]  KtParamMin=[]  KtParamMax=[]  KbOutMin=[]  KbOutMax=[]  KtOutMin=[]  KtOutMax=[]  IntegratorOutMin=[]  IntegratorOutMax=[]  FilterOutMin=[]  FilterOutMax=[]  SumI1OutMin=[]  SumI1OutMax=[]  SumI2OutMin=[]  SumI2OutMax=[]  SumI3OutMin=[]  SumI3OutMax=[]  SumI4OutMin=[]  SumI4OutMax=[]  SumDOutMin=[]  SumDOutMax=[]  Sum1OutMin=[]  Sum1OutMax=[]  Sum2OutMin=[]  Sum2OutMax=[]  Sum3OutMin=[]  Sum3OutMax=[]  DifferentiatorOutMin=[]  DifferentiatorOutMax=[]  FilterDiffOutCoefMin=[]  FilterDiffOutCoefMax=[]  ReciprocalOutMin=[]  ReciprocalOutMax=[]  SumDenOutMin=[]  SumDenOutMax=[]  SumNumOutMin=[]  SumNumOutMax=[]  DivideOutMin=[]  DivideOutMax=[]  UdiffTsProdOutMin=[]  UdiffTsProdOutMax=[]  NTsProdOutMin=[]  NTsProdOutMax=[]  UintegralTsProdOutMin=[]  UintegralTsProdOutMax=[]  UngainTsProdOutMin=[]  UngainTsProdOutMax=[]  ClampingZeroOutDataTypeStr=Inherit: Inherit via back propagation  ClampingZeroOutMin=[]  ClampingZeroOutMax=[]  FilterDenConstantOutDataTypeStr=Inherit: Inherit via back propagation  FilterDenConstantOutMin=[]  FilterDenConstantOutMax=[]  PCopyOutDataTypeStr=Inherit: Inherit via back propagation  PCopyOutMin=[]  PCopyOutMax=[]  NCopyOutDataTypeStr=Inherit: Inherit via back propagation  NCopyOutMin=[]  NCopyOutMax=[]  IntegratorContinuousStateAttributes=''  IntegratorStateMustResolveToSignalObject=off  IntegratorRTWStateStorageClass=Auto  FilterContinuousStateAttributes=''  FilterStateMustResolveToSignalObject=off  FilterRTWStateStorageClass=Auto  ParallelPVariant=InternalParameters  IdealPVariant=Disabled  IVariant=InternalParameters  DVariant=InternalParameters  bVariant=InternalParameters  cVariant=InternalParameters  IntegratorVariant=Continuous  SatVariant=Enabled  AWVariant=ContClampingParallel  PCopyVariant=Disabled  TRVariant=Disabled  FdbkBlocksVariant=Forward  IdealPFdbkVariant=Disabled  SatFdbkVariant=Disabled  DerivativeFilterVariant=ContFilter  NVariant=InternalParameters  NCopyVariant=Disabled  FilterICVariant=InternalICsFilter  IntegratorICVariant=InternalICs  ExternalResetVariant=Disabled  TRSumVariant=Passthrough  SumFdbkVariant=Disabled  SumVariant=Sum_PID  TsampFilterVariant=InternalTs  TsampNgainVariant=Passthrough  TsampIntegralVariant=Disabled_SignalSpec  ExternalSaturationOutDataTypeStr=Inherit: Same as second input
  Bus Selector : BusSelector  OutputSignals=phi
  Constant : Constant  Value=0
  Gain2 : Gain  Gain=-1
  Radians to Degrees : simulink_extras/Transformations/Radians to Degrees
  Lateral Stick : Outport
  Pedal Posn : Outport  Port=2
  " " : Outport  Port=3
  wires:
  BANK HOLD PID/1 -> Gain2/1  "Lat Stick"
  Gain2/1 -> Lateral Stick/1
  Radians to Degrees/1 -> BANK HOLD PID/2
  States/1 -> " "/1, Bus Selector/1
  Bus Selector/1 -> Radians to Degrees/1  "<phi>"
  Reference/1 -> BANK HOLD PID/1
  Constant/1 -> Pedal Posn/1

== system DA40_Flight_Model/Truth Model/Control/Subsystem1 ==
  Reference : Inport
  States : Inport  Port=2
  Bus Selector : BusSelector  OutputSignals=z,theta
  Gain : Gain  Gain=-1
  Gain1 : Gain  Gain=-1
  PID Controller (2DOF)1 : slpidlib/PID Controller (2DOF)  Controller=PID  Form=Parallel  TimeDomain=Continuous-time  UseExternalTs=off  SampleTime=-1  IntegratorMethod=Forward Euler  FilterMethod=Forward Euler  ControllerParametersSource=internal  P=0.392178102036374  I=0.0013184227867295  UseKiTs=off  D=-0.0973934682361479  N=4.02673925817559  UseFilter=on  b=1  c=1  TunerSelectOption=Transfer Function Based (PID Tuner App)  InitialConditionSource=internal  InitialConditionForIntegrator=0  InitialConditionForFilter=0  DifferentiatorICPrevScaledInput=0  ExternalReset=none  TrackingMode=off  Kt=1  LimitOutput=on  SatLimitsSource=internal  UpperSaturationLimit=15  LowerSaturationLimit=-15  LinearizeAsGain=on  AntiWindupMode=clamping  Kb=1  LimitIntegrator=off  UpperIntegratorSaturationLimit=inf  LowerIntegratorSaturationLimit=-inf  POutMin=[]  POutMax=[]  IOutMin=[]  IOutMax=[]  DOutMin=[]  DOutMax=[]  NOutMin=[]  NOutMax=[]  bOutMin=[]  bOutMax=[]  cOutMin=[]  cOutMax=[]  SumOutMin=[]  SumOutMax=[]  SaturationOutMin=[]  SaturationOutMax=[]  PParamMin=[]  PParamMax=[]  IParamMin=[]  IParamMax=[]  DParamMin=[]  DParamMax=[]  NParamMin=[]  NParamMax=[]  bParamMin=[]  bParamMax=[]  cParamMin=[]  cParamMax=[]  KbParamMin=[]  KbParamMax=[]  KtParamMin=[]  KtParamMax=[]  KbOutMin=[]  KbOutMax=[]  KtOutMin=[]  KtOutMax=[]  IntegratorOutMin=[]  IntegratorOutMax=[]  FilterOutMin=[]  FilterOutMax=[]  SumI1OutMin=[]  SumI1OutMax=[]  SumI2OutMin=[]  SumI2OutMax=[]  SumI3OutMin=[]  SumI3OutMax=[]  SumI4OutMin=[]  SumI4OutMax=[]  SumDOutMin=[]  SumDOutMax=[]  Sum1OutMin=[]  Sum1OutMax=[]  Sum2OutMin=[]  Sum2OutMax=[]  Sum3OutMin=[]  Sum3OutMax=[]  DifferentiatorOutMin=[]  DifferentiatorOutMax=[]  FilterDiffOutCoefMin=[]  FilterDiffOutCoefMax=[]  ReciprocalOutMin=[]  ReciprocalOutMax=[]  SumDenOutMin=[]  SumDenOutMax=[]  SumNumOutMin=[]  SumNumOutMax=[]  DivideOutMin=[]  DivideOutMax=[]  UdiffTsProdOutMin=[]  UdiffTsProdOutMax=[]  NTsProdOutMin=[]  NTsProdOutMax=[]  UintegralTsProdOutMin=[]  UintegralTsProdOutMax=[]  UngainTsProdOutMin=[]  UngainTsProdOutMax=[]  ClampingZeroOutDataTypeStr=Inherit: Inherit via back propagation  ClampingZeroOutMin=[]  ClampingZeroOutMax=[]  FilterDenConstantOutDataTypeStr=Inherit: Inherit via back propagation  FilterDenConstantOutMin=[]  FilterDenConstantOutMax=[]  PCopyOutDataTypeStr=Inherit: Inherit via back propagation  PCopyOutMin=[]  PCopyOutMax=[]  NCopyOutDataTypeStr=Inherit: Inherit via back propagation  NCopyOutMin=[]  NCopyOutMax=[]  IntegratorContinuousStateAttributes=''  IntegratorStateMustResolveToSignalObject=off  IntegratorRTWStateStorageClass=Auto  FilterContinuousStateAttributes=''  FilterStateMustResolveToSignalObject=off  FilterRTWStateStorageClass=Auto  ParallelPVariant=InternalParameters  IdealPVariant=Disabled  IVariant=InternalParameters  DVariant=InternalParameters  bVariant=InternalParameters  cVariant=InternalParameters  IntegratorVariant=Continuous  SatVariant=Enabled  AWVariant=ContClampingParallel  PCopyVariant=Disabled  TRVariant=Disabled  FdbkBlocksVariant=Forward  IdealPFdbkVariant=Disabled  SatFdbkVariant=Disabled  DerivativeFilterVariant=ContFilter  NVariant=InternalParameters  NCopyVariant=Disabled  FilterICVariant=InternalICsFilter  IntegratorICVariant=InternalICs  ExternalResetVariant=Disabled  TRSumVariant=Passthrough  SumFdbkVariant=Disabled  SumVariant=Sum_PID  TsampFilterVariant=InternalTs  TsampNgainVariant=Passthrough  TsampIntegralVariant=Disabled_SignalSpec  ExternalSaturationOutDataTypeStr=Inherit: Same as second input
  PITCH HOLD PID : slpidlib/PID Controller (2DOF)  Controller=PID  Form=Parallel  TimeDomain=Continuous-time  UseExternalTs=off  SampleTime=-1  IntegratorMethod=Forward Euler  FilterMethod=Forward Euler  ControllerParametersSource=internal  P=0.06  I=0.01  UseKiTs=off  D=0.02  N=100  UseFilter=on  b=1  c=0  TunerSelectOption=Transfer Function Based (PID Tuner App)  InitialConditionSource=internal  InitialConditionForIntegrator=0  InitialConditionForFilter=0  DifferentiatorICPrevScaledInput=0  ExternalReset=none  TrackingMode=off  Kt=1  LimitOutput=on  SatLimitsSource=internal  UpperSaturationLimit=1  LowerSaturationLimit=-1  LinearizeAsGain=on  AntiWindupMode=clamping  Kb=1  LimitIntegrator=off  UpperIntegratorSaturationLimit=inf  LowerIntegratorSaturationLimit=-inf  POutMin=[]  POutMax=[]  IOutMin=[]  IOutMax=[]  DOutMin=[]  DOutMax=[]  NOutMin=[]  NOutMax=[]  bOutMin=[]  bOutMax=[]  cOutMin=[]  cOutMax=[]  SumOutMin=[]  SumOutMax=[]  SaturationOutMin=[]  SaturationOutMax=[]  PParamMin=[]  PParamMax=[]  IParamMin=[]  IParamMax=[]  DParamMin=[]  DParamMax=[]  NParamMin=[]  NParamMax=[]  bParamMin=[]  bParamMax=[]  cParamMin=[]  cParamMax=[]  KbParamMin=[]  KbParamMax=[]  KtParamMin=[]  KtParamMax=[]  KbOutMin=[]  KbOutMax=[]  KtOutMin=[]  KtOutMax=[]  IntegratorOutMin=[]  IntegratorOutMax=[]  FilterOutMin=[]  FilterOutMax=[]  SumI1OutMin=[]  SumI1OutMax=[]  SumI2OutMin=[]  SumI2OutMax=[]  SumI3OutMin=[]  SumI3OutMax=[]  SumI4OutMin=[]  SumI4OutMax=[]  SumDOutMin=[]  SumDOutMax=[]  Sum1OutMin=[]  Sum1OutMax=[]  Sum2OutMin=[]  Sum2OutMax=[]  Sum3OutMin=[]  Sum3OutMax=[]  DifferentiatorOutMin=[]  DifferentiatorOutMax=[]  FilterDiffOutCoefMin=[]  FilterDiffOutCoefMax=[]  ReciprocalOutMin=[]  ReciprocalOutMax=[]  SumDenOutMin=[]  SumDenOutMax=[]  SumNumOutMin=[]  SumNumOutMax=[]  DivideOutMin=[]  DivideOutMax=[]  UdiffTsProdOutMin=[]  UdiffTsProdOutMax=[]  NTsProdOutMin=[]  NTsProdOutMax=[]  UintegralTsProdOutMin=[]  UintegralTsProdOutMax=[]  UngainTsProdOutMin=[]  UngainTsProdOutMax=[]  ClampingZeroOutDataTypeStr=Inherit: Inherit via back propagation  ClampingZeroOutMin=[]  ClampingZeroOutMax=[]  FilterDenConstantOutDataTypeStr=Inherit: Inherit via back propagation  FilterDenConstantOutMin=[]  FilterDenConstantOutMax=[]  PCopyOutDataTypeStr=Inherit: Inherit via back propagation  PCopyOutMin=[]  PCopyOutMax=[]  NCopyOutDataTypeStr=Inherit: Inherit via back propagation  NCopyOutMin=[]  NCopyOutMax=[]  IntegratorContinuousStateAttributes=''  IntegratorStateMustResolveToSignalObject=off  IntegratorRTWStateStorageClass=Auto  FilterContinuousStateAttributes=''  FilterStateMustResolveToSignalObject=off  FilterRTWStateStorageClass=Auto  ParallelPVariant=InternalParameters  IdealPVariant=Disabled  IVariant=InternalParameters  DVariant=InternalParameters  bVariant=InternalParameters  cVariant=InternalParameters  IntegratorVariant=Continuous  SatVariant=Enabled  AWVariant=ContClampingParallel  PCopyVariant=Disabled  TRVariant=Disabled  FdbkBlocksVariant=Forward  IdealPFdbkVariant=Disabled  SatFdbkVariant=Disabled  DerivativeFilterVariant=ContFilter  NVariant=InternalParameters  NCopyVariant=Disabled  FilterICVariant=InternalICsFilter  IntegratorICVariant=InternalICs  ExternalResetVariant=Disabled  TRSumVariant=Passthrough  SumFdbkVariant=Disabled  SumVariant=Sum_PID  TsampFilterVariant=InternalTs  TsampNgainVariant=Passthrough  TsampIntegralVariant=Disabled_SignalSpec  ExternalSaturationOutDataTypeStr=Inherit: Same as second input
  Radians to Degrees1 : simulink_extras/Transformations/Radians to Degrees
  Longitudinal Stick : Outport
  " " : Outport  Port=2
  wires:
  PID Controller (2DOF)1/1 -> PITCH HOLD PID/1
  Reference/1 -> PID Controller (2DOF)1/1  "altitude command [m]"
  PITCH HOLD PID/1 -> Gain/1  "Long Stick"
  Radians to Degrees1/1 -> PITCH HOLD PID/2
  States/1 -> " "/1, Bus Selector/1
  Gain/1 -> Longitudinal Stick/1
  Gain1/1 -> PID Controller (2DOF)1/2
  Bus Selector/1 -> Gain1/1  "<z>"
  Bus Selector/2 -> Radians to Degrees1/1  "<theta>"

== system DA40_Flight_Model/Truth Model/Control/Subsystem10 ==
  Reference : Inport
  States : Inport  Port=2
  Out1 : Outport
  " " : Outport  Port=2
  wires:
  Reference/1 -> Out1/1
  States/1 -> " "/1

== system DA40_Flight_Model/Truth Model/Control/Subsystem11 ==
  Reference : Inport
  States : Inport  Port=2
  Terminator : Terminator
  Out1 : Outport
  wires:
  Reference/1 -> Out1/1
  States/1 -> Terminator/1

== system DA40_Flight_Model/Truth Model/Control/Subsystem3 ==
  Reference : Inport
  States : Inport  Port=2
  MATLAB Function : MATLAB Function  TreatAsAtomicUnit=on
  PID Controller (2DOF) : slpidlib/PID Controller (2DOF)  Controller=PID  Form=Parallel  TimeDomain=Continuous-time  UseExternalTs=off  SampleTime=-1  IntegratorMethod=Forward Euler  FilterMethod=Forward Euler  ControllerParametersSource=internal  P=0.497904922106352  I=0.0979272469433752  UseKiTs=off  D=-0.183968459268293  N=2.70646894628946  UseFilter=on  b=0.574546090887085  c=0.574546090887085  TunerSelectOption=Transfer Function Based (PID Tuner App)  InitialConditionSource=internal  InitialConditionForIntegrator=0  InitialConditionForFilter=0  DifferentiatorICPrevScaledInput=0  ExternalReset=none  TrackingMode=off  Kt=1  LimitOutput=on  SatLimitsSource=internal  UpperSaturationLimit=1  LowerSaturationLimit=0  LinearizeAsGain=on  AntiWindupMode=none  Kb=1  LimitIntegrator=off  UpperIntegratorSaturationLimit=inf  LowerIntegratorSaturationLimit=-inf  POutMin=[]  POutMax=[]  IOutMin=[]  IOutMax=[]  DOutMin=[]  DOutMax=[]  NOutMin=[]  NOutMax=[]  bOutMin=[]  bOutMax=[]  cOutMin=[]  cOutMax=[]  SumOutMin=[]  SumOutMax=[]  SaturationOutMin=[]  SaturationOutMax=[]  PParamMin=[]  PParamMax=[]  IParamMin=[]  IParamMax=[]  DParamMin=[]  DParamMax=[]  NParamMin=[]  NParamMax=[]  bParamMin=[]  bParamMax=[]  cParamMin=[]  cParamMax=[]  KbParamMin=[]  KbParamMax=[]  KtParamMin=[]  KtParamMax=[]  KbOutMin=[]  KbOutMax=[]  KtOutMin=[]  KtOutMax=[]  IntegratorOutMin=[]  IntegratorOutMax=[]  FilterOutMin=[]  FilterOutMax=[]  SumI1OutMin=[]  SumI1OutMax=[]  SumI2OutMin=[]  SumI2OutMax=[]  SumI3OutMin=[]  SumI3OutMax=[]  SumI4OutMin=[]  SumI4OutMax=[]  SumDOutMin=[]  SumDOutMax=[]  Sum1OutMin=[]  Sum1OutMax=[]  Sum2OutMin=[]  Sum2OutMax=[]  Sum3OutMin=[]  Sum3OutMax=[]  DifferentiatorOutMin=[]  DifferentiatorOutMax=[]  FilterDiffOutCoefMin=[]  FilterDiffOutCoefMax=[]  ReciprocalOutMin=[]  ReciprocalOutMax=[]  SumDenOutMin=[]  SumDenOutMax=[]  SumNumOutMin=[]  SumNumOutMax=[]  DivideOutMin=[]  DivideOutMax=[]  UdiffTsProdOutMin=[]  UdiffTsProdOutMax=[]  NTsProdOutMin=[]  NTsProdOutMax=[]  UintegralTsProdOutMin=[]  UintegralTsProdOutMax=[]  UngainTsProdOutMin=[]  UngainTsProdOutMax=[]  ClampingZeroOutDataTypeStr=Inherit: Inherit via back propagation  ClampingZeroOutMin=[]  ClampingZeroOutMax=[]  FilterDenConstantOutDataTypeStr=Inherit: Inherit via back propagation  FilterDenConstantOutMin=[]  FilterDenConstantOutMax=[]  PCopyOutDataTypeStr=Inherit: Inherit via back propagation  PCopyOutMin=[]  PCopyOutMax=[]  NCopyOutDataTypeStr=Inherit: Inherit via back propagation  NCopyOutMin=[]  NCopyOutMax=[]  IntegratorContinuousStateAttributes=''  IntegratorStateMustResolveToSignalObject=off  IntegratorRTWStateStorageClass=Auto  FilterContinuousStateAttributes=''  FilterStateMustResolveToSignalObject=off  FilterRTWStateStorageClass=Auto  ParallelPVariant=InternalParameters  IdealPVariant=Disabled  IVariant=InternalParameters  DVariant=InternalParameters  bVariant=InternalParameters  cVariant=InternalParameters  IntegratorVariant=Continuous  SatVariant=Enabled  AWVariant=Passthrough  PCopyVariant=Disabled  TRVariant=Disabled  FdbkBlocksVariant=Forward  IdealPFdbkVariant=Disabled  SatFdbkVariant=Disabled  DerivativeFilterVariant=ContFilter  NVariant=InternalParameters  NCopyVariant=Disabled  FilterICVariant=InternalICsFilter  IntegratorICVariant=InternalICs  ExternalResetVariant=Disabled  TRSumVariant=Passthrough  SumFdbkVariant=Disabled  SumVariant=Sum_PID  TsampFilterVariant=InternalTs  TsampNgainVariant=Passthrough  TsampIntegralVariant=Disabled_SignalSpec  ExternalSaturationOutDataTypeStr=Inherit: Same as second input
  Out1 : Outport
  " " : Outport  Port=2
  wires:
  PID Controller (2DOF)/1 -> Out1/1
  States/1 -> " "/1, MATLAB Function/1(X)
  MATLAB Function/1(Aircraft_Airspeed) -> PID Controller (2DOF)/2
  Reference/1 -> PID Controller (2DOF)/1
